simulink model "model_compatible"  (Simulink 7.5)
(part 10 of 10)

  T_173659686_220000_Enichem_Ottana/RConn1 -- L_173659686/LConn1
  T_173659686_220000_Enichem_Ottana/RConn2 -- L_173659686/LConn2
  L_173659686/LConn3 -- T_173659686_220000_Enichem_Ottana/RConn3 -- bus504/LConn1
  T_144006711_220000_Ottana/RConn1 -- L_144006711/LConn1
  T_144006711_220000_Ottana/RConn2 -- L_144006711/LConn2
  L_144006711/LConn3 -- T_144006711_220000_Ottana/RConn3 -- bus505/LConn1
  T_41360305_380000_Poggio_a_Caiano/RConn1 -- L_41360305/LConn1
  T_41360305_380000_Poggio_a_Caiano/RConn2 -- L_41360305/LConn2
  L_41360305/LConn3 -- T_41360305_380000_Poggio_a_Caiano/RConn3 -- bus506/LConn1
  T_139975773_380000_Casellina/RConn1 -- L_139975773/LConn1
  T_139975773_380000_Casellina/RConn2 -- L_139975773/LConn2
  L_139975773/LConn3 -- T_139975773_380000_Casellina/RConn3 -- bus507/LConn1
  T_132455976_220000_Sant'Antimo/RConn1 -- L_132455976/LConn1
  T_132455976_220000_Sant'Antimo/RConn2 -- L_132455976/LConn2
  L_132455976/LConn3 -- T_132455976_220000_Sant'Antimo/RConn3 -- bus508/LConn1
  T_132725149_220000_Astroni/RConn1 -- L_132725149/LConn1
  T_132725149_220000_Astroni/RConn2 -- L_132725149/LConn2
  L_132725149/LConn3 -- T_132725149_220000_Astroni/RConn3 -- bus509/LConn1
  T_132702940_60000;220000_Frattamaggiore/RConn1 -- L_132702940/LConn1
  T_132702940_60000;220000_Frattamaggiore/RConn2 -- L_132702940/LConn2
  L_132702940/LConn3 -- T_132702940_60000;220000_Frattamaggiore/RConn3 -- bus510/LConn1
  T_36873258_380000_Candia/RConn1 -- L_36873258/LConn1
  T_36873258_380000_Candia/RConn2 -- L_36873258/LConn2
  L_36873258/LConn3 -- T_36873258_380000_Candia/RConn3 -- bus511/LConn1
  T_136457747_220000_Abbadia/RConn1 -- L_136457747/LConn1
  T_136457747_220000_Abbadia/RConn2 -- L_136457747/LConn2
  L_136457747/LConn3 -- T_136457747_220000_Abbadia/RConn3 -- bus512/LConn1
  T_158652469_220000_Montorio/RConn1 -- L_158652469/LConn1
  T_158652469_220000_Montorio/RConn2 -- L_158652469/LConn2
  L_158652469/LConn3 -- T_158652469_220000_Montorio/RConn3 -- bus513/LConn1
  T_159821869_220000_Soverzene/RConn1 -- L_159821869/LConn1
  T_159821869_220000_Soverzene/RConn2 -- L_159821869/LConn2
  L_159821869/LConn3 -- T_159821869_220000_Soverzene/RConn3 -- bus514/LConn1
  T_128602121_220000_Scorzè/RConn1 -- L_128602121/LConn1
  T_128602121_220000_Scorzè/RConn2 -- L_128602121/LConn2
  L_128602121/LConn3 -- T_128602121_220000_Scorzè/RConn3 -- bus515/LConn1
  T_155976582_220000_Fadalto/RConn1 -- L_155976582/LConn1
  T_155976582_220000_Fadalto/RConn2 -- L_155976582/LConn2
  L_155976582/LConn3 -- T_155976582_220000_Fadalto/RConn3 -- bus516/LConn1
  T_84963374_220000_Flaminia/RConn1 -- L_84963374/LConn1
  T_84963374_220000_Flaminia/RConn2 -- L_84963374/LConn2
  L_84963374/LConn3 -- T_84963374_220000_Flaminia/RConn3 -- bus517/LConn1
  T_165371026__/RConn1 -- L_165371026/LConn1
  T_165371026__/RConn2 -- L_165371026/LConn2
  L_165371026/LConn3 -- T_165371026__/RConn3 -- bus518/LConn1
  T_105827045_220000_Sant'Antonio/RConn1 -- L_105827045/LConn1
  T_105827045_220000_Sant'Antonio/RConn2 -- L_105827045/LConn2
  L_105827045/LConn3 -- T_105827045_220000_Sant'Antonio/RConn3 -- bus519/LConn1
  T_105801489_220000_Kardaun___Cardano/RConn1 -- L_105801489/LConn1
  T_105801489_220000_Kardaun___Cardano/RConn2 -- L_105801489/LConn2
  L_105801489/LConn3 -- T_105801489_220000_Kardaun___Cardano/RConn3 -- bus520/LConn1
  T_147466201_220000_Santa_Massenza_Centrale/RConn1 -- L_147466201/LConn1
  T_147466201_220000_Santa_Massenza_Centrale/RConn2 -- L_147466201/LConn2
  L_147466201/LConn3 -- T_147466201_220000_Santa_Massenza_Centrale/RConn3 -- bus521/LConn1
  T_166196787_220000_Dalmine_BG/RConn1 -- L_166196787/LConn1
  T_166196787_220000_Dalmine_BG/RConn2 -- L_166196787/LConn2
  L_166196787/LConn3 -- T_166196787_220000_Dalmine_BG/RConn3 -- bus522/LConn1
  T_75378894_380000_Cislago/RConn1 -- L_75378894/LConn1
  T_75378894_380000_Cislago/RConn2 -- L_75378894/LConn2
  L_75378894/LConn3 -- T_75378894_380000_Cislago/RConn3 -- bus523/LConn1
  T_68299044_380000_Brugherio___Smistamento_elettrico_TERNA/RConn1 -- L_68299044/LConn1
  T_68299044_380000_Brugherio___Smistamento_elettrico_TERNA/RConn2 -- L_68299044/LConn2
  L_68299044/LConn3 -- T_68299044_380000_Brugherio___Smistamento_elettrico_TERNA/RConn3 -- bus524/LConn1
  T_103264820_220000_Magenta/RConn1 -- L_103264820/LConn1
  T_103264820_220000_Magenta/RConn2 -- L_103264820/LConn2
  L_103264820/LConn3 -- T_103264820_220000_Magenta/RConn3 -- bus525/LConn1
  T_67461115_220000_Novara_Sud/RConn1 -- L_67461115/LConn1
  T_67461115_220000_Novara_Sud/RConn2 -- L_67461115/LConn2
  L_67461115/LConn3 -- T_67461115_220000_Novara_Sud/RConn3 -- bus526/LConn1
  T_62326314_380000_Baggio/RConn1 -- L_62326314/LConn1
  T_62326314_380000_Baggio/RConn2 -- L_62326314/LConn2
  L_62326314/LConn3 -- T_62326314_380000_Baggio/RConn3 -- bus527/LConn1
  T_104114052_220000_Pallanzeno_1/RConn1 -- L_104114052/LConn1
  T_104114052_220000_Pallanzeno_1/RConn2 -- L_104114052/LConn2
  L_104114052/LConn3 -- T_104114052_220000_Pallanzeno_1/RConn3 -- bus528/LConn1
  T_133601333_220000_Cassano_220/RConn1 -- L_133601333/LConn1
  T_133601333_220000_Cassano_220/RConn2 -- L_133601333/LConn2
  L_133601333/LConn3 -- T_133601333_220000_Cassano_220/RConn3 -- bus529/LConn1
  T_116692433_220000_Brescia_Ricevitrice_Ovest/RConn1 -- L_116692433/LConn1
  T_116692433_220000_Brescia_Ricevitrice_Ovest/RConn2 -- L_116692433/LConn2
  L_116692433/LConn3 -- T_116692433_220000_Brescia_Ricevitrice_Ovest/RConn3 -- bus530/LConn1
  T_135270825_220000_Ricevitrice_Sud_Milano/RConn1 -- L_135270825/LConn1
  T_135270825_220000_Ricevitrice_Sud_Milano/RConn2 -- L_135270825/LConn2
  L_135270825/LConn3 -- T_135270825_220000_Ricevitrice_Sud_Milano/RConn3 -- bus531/LConn1
  T_281091768__Malcontenta/RConn1 -- L_281091768/LConn1
  T_281091768__Malcontenta/RConn2 -- L_281091768/LConn2
  L_281091768/LConn3 -- T_281091768__Malcontenta/RConn3 -- bus532/LConn1
  T_202272734_220000_Castegnero/RConn1 -- L_202272734/LConn1
  T_202272734_220000_Castegnero/RConn2 -- L_202272734/LConn2
  L_202272734/LConn3 -- T_202272734_220000_Castegnero/RConn3 -- bus533/LConn1
  T_59153311_380000_Dolo/RConn1 -- L_59153311/LConn1
  T_59153311_380000_Dolo/RConn2 -- L_59153311/LConn2
  L_59153311/LConn3 -- T_59153311_380000_Dolo/RConn3 -- bus534/LConn1
  T_59026315_380000_Salgareda/RConn1 -- L_59026315/LConn1
  T_59026315_380000_Salgareda/RConn2 -- L_59026315/LConn2
  L_59026315/LConn3 -- T_59026315_380000_Salgareda/RConn3 -- bus535/LConn1
  T_59366523_380000;220000;132000_Stazione_elettrica_di_Camin/RConn4 -- L_59366523/LConn1
  T_59366523_380000;220000;132000_Stazione_elettrica_di_Camin/RConn5 -- L_59366523/LConn2
  L_59366523/LConn3 -- T_59366523_380000;220000;132000_Stazione_elettrica_di_Camin/RConn6 -- bus536/LConn1
  T_144005861_220000_Villasor_Centrale/RConn1 -- L_144005861/LConn1
  T_144005861_220000_Villasor_Centrale/RConn2 -- L_144005861/LConn2
  L_144005861/LConn3 -- T_144005861_220000_Villasor_Centrale/RConn3 -- bus537/LConn1
  T_375892276_220000_Portoscuso/RConn1 -- L_375892276/LConn1
  T_375892276_220000_Portoscuso/RConn2 -- L_375892276/LConn2
  L_375892276/LConn3 -- T_375892276_220000_Portoscuso/RConn3 -- bus538/LConn1
  T_57384507_380000_Chiaramonte_Gulfi/RConn1 -- L_57384507/LConn1
  T_57384507_380000_Chiaramonte_Gulfi/RConn2 -- L_57384507/LConn2
  L_57384507/LConn3 -- T_57384507_380000_Chiaramonte_Gulfi/RConn3 -- bus539/LConn1
  T_57380344_220000_Ragusa/RConn1 -- L_57380344/LConn1
  T_57380344_220000_Ragusa/RConn2 -- L_57380344/LConn2
  L_57380344/LConn3 -- T_57380344_220000_Ragusa/RConn3 -- bus540/LConn1
  T_56984450_220000_Favara/RConn1 -- L_56984450/LConn1
  T_56984450_220000_Favara/RConn2 -- L_56984450/LConn2
  L_56984450/LConn3 -- T_56984450_220000_Favara/RConn3 -- bus541/LConn1
  T_210352188_220000_Ghrighine_Centrale/RConn1 -- L_210352188/LConn1
  T_210352188_220000_Ghrighine_Centrale/RConn2 -- L_210352188/LConn2
  L_210352188/LConn3 -- T_210352188_220000_Ghrighine_Centrale/RConn3 -- bus542/LConn1
  T_210352180_220000_CenTrale_Tirso/RConn1 -- L_210352180/LConn1
  T_210352180_220000_CenTrale_Tirso/RConn2 -- L_210352180/LConn2
  L_210352180/LConn3 -- T_210352180_220000_CenTrale_Tirso/RConn3 -- bus543/LConn1
  T_85196861_380000_Montecorvino/RConn1 -- L_85196861/LConn1
  T_85196861_380000_Montecorvino/RConn2 -- L_85196861/LConn2
  L_85196861/LConn3 -- T_85196861_380000_Montecorvino/RConn3 -- bus544/LConn1
  T_376952616_220000_Nocera/RConn1 -- L_376952616/LConn1
  T_376952616_220000_Nocera/RConn2 -- L_376952616/LConn2
  L_376952616/LConn3 -- T_376952616_220000_Nocera/RConn3 -- bus545/LConn1
  T_124220303_220000_Salerno_Nord/RConn1 -- L_124220303/LConn1
  T_124220303_220000_Salerno_Nord/RConn2 -- L_124220303/LConn2
  L_124220303/LConn3 -- T_124220303_220000_Salerno_Nord/RConn3 -- bus546/LConn1
  T_420698910_220000_Tusciano/RConn1 -- L_420698910/LConn1
  T_420698910_220000_Tusciano/RConn2 -- L_420698910/LConn2
  L_420698910/LConn3 -- T_420698910_220000_Tusciano/RConn3 -- bus547/LConn1
  T_85297730_220000_Gragnano/RConn1 -- L_85297730/LConn1
  T_85297730_220000_Gragnano/RConn2 -- L_85297730/LConn2
  L_85297730/LConn3 -- T_85297730_220000_Gragnano/RConn3 -- bus548/LConn1
  T_147455038_220000_Santa_Massenza_Smistamento/RConn1 -- L_147455038/LConn1
  T_147455038_220000_Santa_Massenza_Smistamento/RConn2 -- L_147455038/LConn2
  L_147455038/LConn3 -- T_147455038_220000_Santa_Massenza_Smistamento/RConn3 -- bus549/LConn1
  T_156001963_220000_Stazione_elettrica_di_Sandrà/RConn1 -- L_156001963/LConn1
  T_156001963_220000_Stazione_elettrica_di_Sandrà/RConn2 -- L_156001963/LConn2
  L_156001963/LConn3 -- T_156001963_220000_Stazione_elettrica_di_Sandrà/RConn3 -- bus550/LConn1
  T_132638645_220000_Brusciano/RConn1 -- L_132638645/LConn1
  T_132638645_220000_Brusciano/RConn2 -- L_132638645/LConn2
  L_132638645/LConn3 -- T_132638645_220000_Brusciano/RConn3 -- bus551/LConn1
  T_202711181_220000_Nola/RConn1 -- L_202711181/LConn1
  T_202711181_220000_Nola/RConn2 -- L_202711181/LConn2
  L_202711181/LConn3 -- T_202711181_220000_Nola/RConn3 -- bus552/LConn1
  T_132637884_220000_Fiat_Auto/RConn1 -- L_132637884/LConn1
  T_132637884_220000_Fiat_Auto/RConn2 -- L_132637884/LConn2
  L_132637884/LConn3 -- T_132637884_220000_Fiat_Auto/RConn3 -- bus553/LConn1
  T_132638412__/RConn1 -- L_132638412/LConn1
  T_132638412__/RConn2 -- L_132638412/LConn2
  L_132638412/LConn3 -- T_132638412__/RConn3 -- bus554/LConn1
  T_132701023_220000_Acerra_smistamento/RConn1 -- L_132701023/LConn1
  T_132701023_220000_Acerra_smistamento/RConn2 -- L_132701023/LConn2
  L_132701023/LConn3 -- T_132701023_220000_Acerra_smistamento/RConn3 -- bus555/LConn1
  T_132717802_220000_Maddaloni/RConn1 -- L_132717802/LConn1
  T_132717802_220000_Maddaloni/RConn2 -- L_132717802/LConn2
  L_132717802/LConn3 -- T_132717802_220000_Maddaloni/RConn3 -- bus556/LConn1
  T_163789376_220000_Venina/RConn1 -- L_163789376/LConn1
  T_163789376_220000_Venina/RConn2 -- L_163789376/LConn2
  L_163789376/LConn3 -- T_163789376_220000_Venina/RConn3 -- bus557/LConn1
  T_75947658_220000_Cassano_CS/RConn1 -- L_75947658/LConn1
  T_75947658_220000_Cassano_CS/RConn2 -- L_75947658/LConn2
  L_75947658/LConn3 -- T_75947658_220000_Cassano_CS/RConn3 -- bus558/LConn1
  T_114659171_220000_/RConn1 -- L_114659171/LConn1
  T_114659171_220000_/RConn2 -- L_114659171/LConn2
  L_114659171/LConn3 -- T_114659171_220000_/RConn3 -- bus559/LConn1
  T_318173253__/RConn1 -- L_318173253/LConn1
  T_318173253__/RConn2 -- L_318173253/LConn2
  L_318173253/LConn3 -- T_318173253__/RConn3 -- bus560/LConn1
  T_163056526_220000_Lanzada/RConn1 -- L_163056526/LConn1
  T_163056526_220000_Lanzada/RConn2 -- L_163056526/LConn2
  L_163056526/LConn3 -- T_163056526_220000_Lanzada/RConn3 -- bus561/LConn1
  T_163056522_220000_Sondrio/RConn1 -- L_163056522/LConn1
  T_163056522_220000_Sondrio/RConn2 -- L_163056522/LConn2
  L_163056522/LConn3 -- T_163056522_220000_Sondrio/RConn3 -- bus562/LConn1
  T_59629638_220000_Erzelli/RConn1 -- L_59629638/LConn1
  T_59629638_220000_Erzelli/RConn2 -- L_59629638/LConn2
  L_59629638/LConn3 -- T_59629638_220000_Erzelli/RConn3 -- bus563/LConn1
  T_61484190_220000_Morigallo/RConn1 -- L_61484190/LConn1
  T_61484190_220000_Morigallo/RConn2 -- L_61484190/LConn2
  L_61484190/LConn3 -- T_61484190_220000_Morigallo/RConn3 -- bus564/LConn1
  T_376952589_220000_/RConn1 -- L_376952589/LConn1
  T_376952589_220000_/RConn2 -- L_376952589/LConn2
  L_376952589/LConn3 -- T_376952589_220000_/RConn3 -- bus565/LConn1
  T_370679021_220000_Casalnuovo/RConn1 -- L_370679021/LConn1
  T_370679021_220000_Casalnuovo/RConn2 -- L_370679021/LConn2
  L_370679021/LConn3 -- T_370679021_220000_Casalnuovo/RConn3 -- bus566/LConn1
  T_376952600_220000_Alfa_Avio/RConn1 -- L_376952600/LConn1
  T_376952600_220000_Alfa_Avio/RConn2 -- L_376952600/LConn2
  L_376952600/LConn3 -- T_376952600_220000_Alfa_Avio/RConn3 -- bus567/LConn1
  T_199886416_220000_Mercure/RConn1 -- L_199886416/LConn1
  T_199886416_220000_Mercure/RConn2 -- L_199886416/LConn2
  L_199886416/LConn3 -- T_199886416_220000_Mercure/RConn3 -- bus568/LConn1
  T_108020695_220000_Rotonda/RConn1 -- L_108020695/LConn1
  T_108020695_220000_Rotonda/RConn2 -- L_108020695/LConn2
  L_108020695/LConn3 -- T_108020695_220000_Rotonda/RConn3 -- bus569/LConn1
  T_129407370_220000_Stazione_IV/RConn1 -- L_129407370/LConn1
  T_129407370_220000_Stazione_IV/RConn2 -- L_129407370/LConn2
  L_129407370/LConn3 -- T_129407370_220000_Stazione_IV/RConn3 -- bus570/LConn1
  T_416679117_220000_Villabona/RConn1 -- L_416679117/LConn1
  T_416679117_220000_Villabona/RConn2 -- L_416679117/LConn2
  L_416679117/LConn3 -- T_416679117_220000_Villabona/RConn3 -- bus571/LConn1
  T_129406824_220000;132000_Azotati/RConn1 -- L_129406824/LConn1
  T_129406824_220000;132000_Azotati/RConn2 -- L_129406824/LConn2
  L_129406824/LConn3 -- T_129406824_220000;132000_Azotati/RConn3 -- bus572/LConn1
  T_61650514_220000_Somplago_centrale/RConn1 -- L_61650514/LConn1
  T_61650514_220000_Somplago_centrale/RConn2 -- L_61650514/LConn2
  L_61650514/LConn3 -- T_61650514_220000_Somplago_centrale/RConn3 -- bus573/LConn1
  T_149188707_220000_Cittadella/RConn1 -- L_149188707/LConn1
  T_149188707_220000_Cittadella/RConn2 -- L_149188707/LConn2
  L_149188707/LConn3 -- T_149188707_220000_Cittadella/RConn3 -- bus574/LConn1
  T_128523865_220000_Acciaierie_Venete_220/RConn1 -- L_128523865/LConn1
  T_128523865_220000_Acciaierie_Venete_220/RConn2 -- L_128523865/LConn2
  L_128523865/LConn3 -- T_128523865_220000_Acciaierie_Venete_220/RConn3 -- bus575/LConn1
  T_105062415_220000_Pianezza/RConn1 -- L_105062415/LConn1
  T_105062415_220000_Pianezza/RConn2 -- L_105062415/LConn2
  L_105062415/LConn3 -- T_105062415_220000_Pianezza/RConn3 -- bus576/LConn1
  T_58516664_220000_Martinetto/RConn1 -- L_58516664/LConn1
  T_58516664_220000_Martinetto/RConn2 -- L_58516664/LConn2
  L_58516664/LConn3 -- T_58516664_220000_Martinetto/RConn3 -- bus577/LConn1
  T_105141350_220000_Grugliasco/RConn1 -- L_105141350/LConn1
  T_105141350_220000_Grugliasco/RConn2 -- L_105141350/LConn2
  L_105141350/LConn3 -- T_105141350_220000_Grugliasco/RConn3 -- bus578/LConn1
  T_66872608_220000_Rosone/RConn1 -- L_66872608/LConn1
  T_66872608_220000_Rosone/RConn2 -- L_66872608/LConn2
  L_66872608/LConn3 -- T_66872608_220000_Rosone/RConn3 -- bus579/LConn1
  T_98902899_380000_Piossasco/RConn1 -- L_98902899/LConn1
  T_98902899_380000_Piossasco/RConn2 -- L_98902899/LConn2
  L_98902899/LConn3 -- T_98902899_380000_Piossasco/RConn3 -- bus580/LConn1
  T_163958919_220000_Lambrate/RConn1 -- L_163958919/LConn1
  T_163958919_220000_Lambrate/RConn2 -- L_163958919/LConn2
  L_163958919/LConn3 -- T_163958919_220000_Lambrate/RConn3 -- bus581/LConn1
  T_203771704_220000_UT_CESI/RConn1 -- L_203771704/LConn1
  T_203771704_220000_UT_CESI/RConn2 -- L_203771704/LConn2
  L_203771704/LConn3 -- T_203771704_220000_UT_CESI/RConn3 -- bus582/LConn1
  T_173999201_220000_Napoli_Levante/RConn1 -- L_173999201/LConn1
  T_173999201_220000_Napoli_Levante/RConn2 -- L_173999201/LConn2
  L_173999201/LConn3 -- T_173999201_220000_Napoli_Levante/RConn3 -- bus583/LConn1
  T_376502734_220000_Casoria/RConn1 -- L_376502734/LConn1
  T_376502734_220000_Casoria/RConn2 -- L_376502734/LConn2
  L_376502734/LConn3 -- T_376502734_220000_Casoria/RConn3 -- bus584/LConn1
  T_377444648_220000_/RConn1 -- L_377444648/LConn1
  T_377444648_220000_/RConn2 -- L_377444648/LConn2
  L_377444648/LConn3 -- T_377444648_220000_/RConn3 -- bus585/LConn1
  T_80442466_220000_Grosio/RConn1 -- L_80442466/LConn1
  T_80442466_220000_Grosio/RConn2 -- L_80442466/LConn2
  L_80442466/LConn3 -- T_80442466_220000_Grosio/RConn3 -- bus586/LConn1
  T_165503884_220000_Grosotto/RConn1 -- L_165503884/LConn1
  T_165503884_220000_Grosotto/RConn2 -- L_165503884/LConn2
  L_165503884/LConn3 -- T_165503884_220000_Grosotto/RConn3 -- bus587/LConn1
  T_105757795_220000_Campochiesa/RConn1 -- L_105757795/LConn1
  T_105757795_220000_Campochiesa/RConn2 -- L_105757795/LConn2
  L_105757795/LConn3 -- T_105757795_220000_Campochiesa/RConn3 -- bus588/LConn1
  T_103653567_220000_centrale_elettrica_di_Camporosso/RConn1 -- L_103653567/LConn1
  T_103653567_220000_centrale_elettrica_di_Camporosso/RConn2 -- L_103653567/LConn2
  L_103653567/LConn3 -- T_103653567_220000_centrale_elettrica_di_Camporosso/RConn3 -- bus589/LConn1
  T_309371153_220000_TO_Sud/RConn1 -- L_309371153/LConn1
  T_309371153_220000_TO_Sud/RConn2 -- L_309371153/LConn2
  L_309371153/LConn3 -- T_309371153_220000_TO_Sud/RConn3 -- bus590/LConn1
  T_309371152_220000_TO_Centro/RConn1 -- L_309371152/LConn1
  T_309371152_220000_TO_Centro/RConn2 -- L_309371152/LConn2
  L_309371152/LConn3 -- T_309371152_220000_TO_Centro/RConn3 -- bus591/LConn1
  T_350356755_220000_Colorno/RConn1 -- L_350356755/LConn1
  T_350356755_220000_Colorno/RConn2 -- L_350356755/LConn2
  L_350356755/LConn3 -- T_350356755_220000_Colorno/RConn3 -- bus592/LConn1
  T_163058980_220000_Marcaria/RConn1 -- L_163058980/LConn1
  T_163058980_220000_Marcaria/RConn2 -- L_163058980/LConn2
  L_163058980/LConn3 -- T_163058980_220000_Marcaria/RConn3 -- bus593/LConn1
  T_191960170_220000_Corriolo/RConn1 -- L_191960170/LConn1
  T_191960170_220000_Corriolo/RConn2 -- L_191960170/LConn2
  L_191960170/LConn3 -- T_191960170_220000_Corriolo/RConn3 -- bus594/LConn1
  T_57736553_220000_Caracoli/RConn1 -- L_57736553/LConn1
  T_57736553_220000_Caracoli/RConn2 -- L_57736553/LConn2
  L_57736553/LConn3 -- T_57736553_220000_Caracoli/RConn3 -- bus595/LConn1
  T_136626367__/RConn1 -- L_136626367/LConn1
  T_136626367__/RConn2 -- L_136626367/LConn2
  L_136626367/LConn3 -- T_136626367__/RConn3 -- bus596/LConn1
  T_375892275_220000_Eurallumina/RConn1 -- L_375892275/LConn1
  T_375892275_220000_Eurallumina/RConn2 -- L_375892275/LConn2
  L_375892275/LConn3 -- T_375892275_220000_Eurallumina/RConn3 -- bus597/LConn1
  T_375892277_220000_Samim/RConn1 -- L_375892277/LConn1
  T_375892277_220000_Samim/RConn2 -- L_375892277/LConn2
  L_375892277/LConn3 -- T_375892277_220000_Samim/RConn3 -- bus598/LConn1
  T_375892272_220000_Samim/RConn1 -- L_375892272/LConn1
  T_375892272_220000_Samim/RConn2 -- L_375892272/LConn2
  L_375892272/LConn3 -- T_375892272_220000_Samim/RConn3 -- bus599/LConn1
  T_107204719_220000_Tavazzano_Est/RConn1 -- L_107204719/LConn1
  T_107204719_220000_Tavazzano_Est/RConn2 -- L_107204719/LConn2
  L_107204719/LConn3 -- T_107204719_220000_Tavazzano_Est/RConn3 -- bus600/LConn1
  T_74359510_220000_Cesano_Maderno/RConn1 -- L_74359510/LConn1
  T_74359510_220000_Cesano_Maderno/RConn2 -- L_74359510/LConn2
  L_74359510/LConn3 -- T_74359510_220000_Cesano_Maderno/RConn3 -- bus601/LConn1
  T_156001981_220000_Colà/RConn1 -- L_156001981/LConn1
  T_156001981_220000_Colà/RConn2 -- L_156001981/LConn2
  L_156001981/LConn3 -- T_156001981_220000_Colà/RConn3 -- bus602/LConn1
  T_116916459_220000_Tavazzano_ST/RConn1 -- L_116916459/LConn1
  T_116916459_220000_Tavazzano_ST/RConn2 -- L_116916459/LConn2
  L_116916459/LConn3 -- T_116916459_220000_Tavazzano_ST/RConn3 -- bus603/LConn1
  T_60725872_380000_Monfalcone_sezione_1_220/LConn1 -- L_60725872/LConn1
  T_60725872_380000_Monfalcone_sezione_1_220/LConn2 -- L_60725872/LConn2
  L_60725872/LConn3 -- T_60725872_380000_Monfalcone_sezione_1_220/LConn3 -- bus604/LConn1
  T_41892273_380000_Redipuglia/RConn1 -- L_41892273/LConn1
  T_41892273_380000_Redipuglia/RConn2 -- L_41892273/LConn2
  L_41892273/LConn3 -- T_41892273_380000_Redipuglia/RConn3 -- bus605/LConn1
  T_61038773_220000_Padriciano/RConn1 -- L_61038773/LConn1
  T_61038773_220000_Padriciano/RConn2 -- L_61038773/LConn2
  L_61038773/LConn3 -- T_61038773_220000_Padriciano/RConn3 -- bus606/LConn1
  T_105141365_380000_Laboratori_Cesi_Chivasso/RConn1 -- L_105141365/LConn1
  T_105141365_380000_Laboratori_Cesi_Chivasso/RConn2 -- L_105141365/LConn2
  L_105141365/LConn3 -- T_105141365_380000_Laboratori_Cesi_Chivasso/RConn3 -- bus607/LConn1
  T_82651599_220000_Biella_Est/RConn1 -- L_82651599/LConn1
  T_82651599_220000_Biella_Est/RConn2 -- L_82651599/LConn2
  L_82651599/LConn3 -- T_82651599_220000_Biella_Est/RConn3 -- bus608/LConn1
  T_74869121_380000_Rondissone/RConn1 -- L_74869121/LConn1
  T_74869121_380000_Rondissone/RConn2 -- L_74869121/LConn2
  L_74869121/LConn3 -- T_74869121_380000_Rondissone/RConn3 -- bus609/LConn1
  T_103725268_220000_Stura/RConn1 -- L_103725268/LConn1
  T_103725268_220000_Stura/RConn2 -- L_103725268/LConn2
  L_103725268/LConn3 -- T_103725268_220000_Stura/RConn3 -- bus610/LConn1
  T_100952845_380000_Vignole/RConn1 -- L_100952845/LConn1
  T_100952845_380000_Vignole/RConn2 -- L_100952845/LConn2
  L_100952845/LConn3 -- T_100952845_380000_Vignole/RConn3 -- bus611/LConn1
  T_79879290_220000_Ricevitrice_Nord_Milano/RConn1 -- L_79879290/LConn1
  T_79879290_220000_Ricevitrice_Nord_Milano/RConn2 -- L_79879290/LConn2
  L_79879290/LConn3 -- T_79879290_220000_Ricevitrice_Nord_Milano/RConn3 -- bus612/LConn1
  T_146652798_220000_Centro_Energia_Teverola/RConn1 -- L_146652798/LConn1
  T_146652798_220000_Centro_Energia_Teverola/RConn2 -- L_146652798/LConn2
  L_146652798/LConn3 -- T_146652798_220000_Centro_Energia_Teverola/RConn3 -- bus613/LConn1
  T_132701980_220000_Aversa/RConn1 -- L_132701980/LConn1
  T_132701980_220000_Aversa/RConn2 -- L_132701980/LConn2
  L_132701980/LConn3 -- T_132701980_220000_Aversa/RConn3 -- bus614/LConn1
  T_96658563_220000_Lavis/RConn1 -- L_96658563/LConn1
  T_96658563_220000_Lavis/RConn2 -- L_96658563/LConn2
  L_96658563/LConn3 -- T_96658563_220000_Lavis/RConn3 -- bus615/LConn1
  T_103549584_220000_Borgo_Valsugana/RConn1 -- L_103549584/LConn1
  T_103549584_220000_Borgo_Valsugana/RConn2 -- L_103549584/LConn2
  L_103549584/LConn3 -- T_103549584_220000_Borgo_Valsugana/RConn3 -- bus616/LConn1
  T_151070909_220000_San_Floriano_d'Egna/RConn1 -- L_151070909/LConn1
  T_151070909_220000_San_Floriano_d'Egna/RConn2 -- L_151070909/LConn2
  L_151070909/LConn3 -- T_151070909_220000_San_Floriano_d'Egna/RConn3 -- bus617/LConn1
  T_419423704_220000_Presenzano_TR/RConn1 -- L_419423704/LConn1
  T_419423704_220000_Presenzano_TR/RConn2 -- L_419423704/LConn2
  L_419423704/LConn3 -- T_419423704_220000_Presenzano_TR/RConn3 -- bus618/LConn1
  T_93860115_380000_Santa_Maria_Capua_Vetere/RConn1 -- L_93860115/LConn1
  T_93860115_380000_Santa_Maria_Capua_Vetere/RConn2 -- L_93860115/LConn2
  L_93860115/LConn3 -- T_93860115_380000_Santa_Maria_Capua_Vetere/RConn3 -- bus619/LConn1
  T_202772821_220000_Ganda/RConn1 -- L_202772821/LConn1
  T_202772821_220000_Ganda/RConn2 -- L_202772821/LConn2
  L_202772821/LConn3 -- T_202772821_220000_Ganda/RConn3 -- bus620/LConn1
  T_61375111_380000_Villanova/RConn1 -- L_61375111/LConn1
  T_61375111_380000_Villanova/RConn2 -- L_61375111/LConn2
  L_61375111/LConn3 -- T_61375111_380000_Villanova/RConn3 -- bus621/LConn1
  T_139758444_220000_Querceto/RConn1 -- L_139758444/LConn1
  T_139758444_220000_Querceto/RConn2 -- L_139758444/LConn2
  L_139758444/LConn3 -- T_139758444_220000_Querceto/RConn3 -- bus622/LConn1
  T_139442467_380000_Colunga/RConn1 -- L_139442467/LConn1
  T_139442467_380000_Colunga/RConn2 -- L_139442467/LConn2
  L_139442467/LConn3 -- T_139442467_380000_Colunga/RConn3 -- bus623/LConn1
  T_40634284_380000_Calenzano/RConn1 -- L_40634284/LConn1
  T_40634284_380000_Calenzano/RConn2 -- L_40634284/LConn2
  L_40634284/LConn3 -- T_40634284_380000_Calenzano/RConn3 -- bus624/LConn1
  T_107241327_220000_Tavazzano_Ovest/RConn1 -- L_107241327/LConn1
  T_107241327_220000_Tavazzano_Ovest/RConn2 -- L_107241327/LConn2
  L_107241327/LConn3 -- T_107241327_220000_Tavazzano_Ovest/RConn3 -- bus625/LConn1
  T_203468251_220000;132000_RISE_Sesto/RConn1 -- L_203468251/LConn1
  T_203468251_220000;132000_RISE_Sesto/RConn2 -- L_203468251/LConn2
  L_203468251/LConn3 -- T_203468251_220000;132000_RISE_Sesto/RConn3 -- bus626/LConn1
  T_93850768_220000_Castelluccia/RConn1 -- L_93850768/LConn1
  T_93850768_220000_Castelluccia/RConn2 -- L_93850768/LConn2
  L_93850768/LConn3 -- T_93850768_220000_Castelluccia/RConn3 -- bus627/LConn1
  T_202179289_220000_/RConn1 -- L_202179289/LConn1
  T_202179289_220000_/RConn2 -- L_202179289/LConn2
  L_202179289/LConn3 -- T_202179289_220000_/RConn3 -- bus628/LConn1
  T_59604857_220000_Acciaieria_Bertoli/RConn1 -- L_59604857/LConn1
  T_59604857_220000_Acciaieria_Bertoli/RConn2 -- L_59604857/LConn2
  L_59604857/LConn3 -- T_59604857_220000_Acciaieria_Bertoli/RConn3 -- bus629/LConn1
  T_165371027__/RConn1 -- L_165371027/LConn1
  T_165371027__/RConn2 -- L_165371027/LConn2
  L_165371027/LConn3 -- T_165371027__/RConn3 -- bus630/LConn1
  T_82762493_380000_Santa_Lucia/RConn1 -- L_82762493/LConn1
  T_82762493_380000_Santa_Lucia/RConn2 -- L_82762493/LConn2
  L_82762493/LConn3 -- T_82762493_380000_Santa_Lucia/RConn3 -- bus631/LConn1
  T_151205012_220000_Boazzo/RConn1 -- L_151205012/LConn1
  T_151205012_220000_Boazzo/RConn2 -- L_151205012/LConn2
  L_151205012/LConn3 -- T_151205012_220000_Boazzo/RConn3 -- bus632/LConn1
  T_151199514_220000_Cimego_TR/RConn1 -- L_151199514/LConn1
  T_151199514_220000_Cimego_TR/RConn2 -- L_151199514/LConn2
  L_151199514/LConn3 -- T_151199514_220000_Cimego_TR/RConn3 -- bus633/LConn1
  T_103653565_220000_San_Colombano/RConn1 -- L_103653565/LConn1
  T_103653565_220000_San_Colombano/RConn2 -- L_103653565/LConn2
  L_103653565/LConn3 -- T_103653565_220000_San_Colombano/RConn3 -- bus634/LConn1
  T_158599954_220000_Stazione_elettrica_di_Avenza/RConn1 -- L_158599954/LConn1
  T_158599954_220000_Stazione_elettrica_di_Avenza/RConn2 -- L_158599954/LConn2
  L_158599954/LConn3 -- T_158599954_220000_Stazione_elettrica_di_Avenza/RConn3 -- bus635/LConn1
  T_296141722_220000_Savona_T5/RConn1 -- L_296141722/LConn1
  T_296141722_220000_Savona_T5/RConn2 -- L_296141722/LConn2
  L_296141722/LConn3 -- T_296141722_220000_Savona_T5/RConn3 -- bus636/LConn1
  T_375908008_220000_Fulgatore/RConn1 -- L_375908008/LConn1
  T_375908008_220000_Fulgatore/RConn2 -- L_375908008/LConn2
  L_375908008/LConn3 -- T_375908008_220000_Fulgatore/RConn3 -- bus637/LConn1
  T_53635045__Partanna/RConn1 -- L_53635045/LConn1
  T_53635045__Partanna/RConn2 -- L_53635045/LConn2
  L_53635045/LConn3 -- T_53635045__Partanna/RConn3 -- bus638/LConn1
  T_110140586_220000_San_Filippo_del_Mela_gruppi_5_e_6/RConn1 -- L_110140586/LConn1
  T_110140586_220000_San_Filippo_del_Mela_gruppi_5_e_6/RConn2 -- L_110140586/LConn2
  L_110140586/LConn3 -- T_110140586_220000_San_Filippo_del_Mela_gruppi_5_e_6/RConn3 -- bus639/LConn1
  T_111020792_220000_Stazione_elettrica_di_Bussolengo/RConn1 -- L_111020792/LConn1
  T_111020792_220000_Stazione_elettrica_di_Bussolengo/RConn2 -- L_111020792/LConn2
  L_111020792/LConn3 -- T_111020792_220000_Stazione_elettrica_di_Bussolengo/RConn3 -- bus640/LConn1
  T_59556712_380000_Dugale/RConn1 -- L_59556712/LConn1
  T_59556712_380000_Dugale/RConn2 -- L_59556712/LConn2
  L_59556712/LConn3 -- T_59556712_380000_Dugale/RConn3 -- bus641/LConn1
  T_412909650_220000_Mantova_220/RConn1 -- L_412909650/LConn1
  T_412909650_220000_Mantova_220/RConn2 -- L_412909650/LConn2
  L_412909650/LConn3 -- T_412909650_220000_Mantova_220/RConn3 -- bus642/LConn1
  T_155976563_220000_Conegliano/RConn1 -- L_155976563/LConn1
  T_155976563_220000_Conegliano/RConn2 -- L_155976563/LConn2
  L_155976563/LConn3 -- T_155976563_220000_Conegliano/RConn3 -- bus643/LConn1
  T_96188601_220000_San_Giacomo_220/RConn1 -- L_96188601/LConn1
  T_96188601_220000_San_Giacomo_220/RConn2 -- L_96188601/LConn2
  L_96188601/LConn3 -- T_96188601_220000_San_Giacomo_220/RConn3 -- bus644/LConn1
  T_84277460_220000_Popoli/RConn1 -- L_84277460/LConn1
  T_84277460_220000_Popoli/RConn2 -- L_84277460/LConn2
  L_84277460/LConn3 -- T_84277460_220000_Popoli/RConn3 -- bus645/LConn1
  T_96190189_380000_San_Giacomo_380/RConn1 -- L_96190189/LConn1
  T_96190189_380000_San_Giacomo_380/RConn2 -- L_96190189/LConn2
  L_96190189/LConn3 -- T_96190189_380000_San_Giacomo_380/RConn3 -- bus646/LConn1
  T_108020416_380000_Laino/RConn1 -- L_108020416/LConn1
  T_108020416_380000_Laino/RConn2 -- L_108020416/LConn2
  L_108020416/LConn3 -- T_108020416_380000_Laino/RConn3 -- bus647/LConn1
  T_144378054_220000_Arezzo_C/RConn1 -- L_144378054/LConn1
  T_144378054_220000_Arezzo_C/RConn2 -- L_144378054/LConn2
  L_144378054/LConn3 -- T_144378054_220000_Arezzo_C/RConn3 -- bus648/LConn1
  T_120916823_220000_Pietrafitta_220/RConn1 -- L_120916823/LConn1
  T_120916823_220000_Pietrafitta_220/RConn2 -- L_120916823/LConn2
  L_120916823/LConn3 -- T_120916823_220000_Pietrafitta_220/RConn3 -- bus649/LConn1
  T_59620552_220000_Naturno/RConn1 -- L_59620552/LConn1
  T_59620552_220000_Naturno/RConn2 -- L_59620552/LConn2
  L_59620552/LConn3 -- T_59620552_220000_Naturno/RConn3 -- bus650/LConn1
  T_35680992_220000_Ponte_Resia/RConn1 -- L_35680992/LConn1
  T_35680992_220000_Ponte_Resia/RConn2 -- L_35680992/LConn2
  L_35680992/LConn3 -- T_35680992_220000_Ponte_Resia/RConn3 -- bus651/LConn1
  T_101346507_220000_Novi_Ligure/RConn1 -- L_101346507/LConn1
  T_101346507_220000_Novi_Ligure/RConn2 -- L_101346507/LConn2
  L_101346507/LConn3 -- T_101346507_220000_Novi_Ligure/RConn3 -- bus652/LConn1
  T_101346508_220000_Ital_Novi/RConn1 -- L_101346508/LConn1
  T_101346508_220000_Ital_Novi/RConn2 -- L_101346508/LConn2
  L_101346508/LConn3 -- T_101346508_220000_Ital_Novi/RConn3 -- bus653/LConn1
  T_95466193_220000_/RConn1 -- L_95466193/LConn1
  T_95466193_220000_/RConn2 -- L_95466193/LConn2
  L_95466193/LConn3 -- T_95466193_220000_/RConn3 -- bus654/LConn1
  T_76705565_380000;220000;150000_Roma_Sud/RConn4 -- L_76705565/LConn1
  T_76705565_380000;220000;150000_Roma_Sud/RConn5 -- L_76705565/LConn2
  L_76705565/LConn3 -- T_76705565_380000;220000;150000_Roma_Sud/RConn6 -- bus655/LConn1
  T_375916035_220000_Cattolica_Eraclea_centrale/RConn1 -- L_375916035/LConn1
  T_375916035_220000_Cattolica_Eraclea_centrale/RConn2 -- L_375916035/LConn2
  L_375916035/LConn3 -- T_375916035_220000_Cattolica_Eraclea_centrale/RConn3 -- bus656/LConn1
  T_375907988_220000_Sambuca/RConn1 -- L_375907988/LConn1
  T_375907988_220000_Sambuca/RConn2 -- L_375907988/LConn2
  L_375907988/LConn3 -- T_375907988_220000_Sambuca/RConn3 -- bus657/LConn1
  T_132726160_220000_Pozzuoli/RConn1 -- L_132726160/LConn1
  T_132726160_220000_Pozzuoli/RConn2 -- L_132726160/LConn2
  L_132726160/LConn3 -- T_132726160_220000_Pozzuoli/RConn3 -- bus658/LConn1
  T_377832777_220000_Tirano/RConn1 -- L_377832777/LConn1
  T_377832777_220000_Tirano/RConn2 -- L_377832777/LConn2
  L_377832777/LConn3 -- T_377832777_220000_Tirano/RConn3 -- bus659/LConn1
  T_98787157_220000_Glorenza/RConn1 -- L_98787157/LConn1
  T_98787157_220000_Glorenza/RConn2 -- L_98787157/LConn2
  L_98787157/LConn3 -- T_98787157_220000_Glorenza/RConn3 -- bus660/LConn1
  T_377588184_220000_Caivano/RConn1 -- L_377588184/LConn1
  T_377588184_220000_Caivano/RConn2 -- L_377588184/LConn2
  L_377588184/LConn3 -- T_377588184_220000_Caivano/RConn3 -- bus661/LConn1
  T_132719324_220000_Air_Liquide/RConn1 -- L_132719324/LConn1
  T_132719324_220000_Air_Liquide/RConn2 -- L_132719324/LConn2
  L_132719324/LConn3 -- T_132719324_220000_Air_Liquide/RConn3 -- bus662/LConn1
  T_84696559_380000_Santa_Sofia/RConn1 -- L_84696559/LConn1
  T_84696559_380000_Santa_Sofia/RConn2 -- L_84696559/LConn2
  L_84696559/LConn3 -- T_84696559_380000_Santa_Sofia/RConn3 -- bus663/LConn1
  T_162960205_380000_Tavazzano_Centrale/RConn1 -- L_162960205/LConn1
  T_162960205_380000_Tavazzano_Centrale/RConn2 -- L_162960205/LConn2
  L_162960205/LConn3 -- T_162960205_380000_Tavazzano_Centrale/RConn3 -- bus664/LConn1
  T_214294769_220000_Moline/RConn1 -- L_214294769/LConn1
  T_214294769_220000_Moline/RConn2 -- L_214294769/LConn2
  L_214294769/LConn3 -- T_214294769_220000_Moline/RConn3 -- bus665/LConn1
  T_281837810_220000_Cedegolo_Sud/RConn1 -- L_281837810/LConn1
  T_281837810_220000_Cedegolo_Sud/RConn2 -- L_281837810/LConn2
  L_281837810/LConn3 -- T_281837810_220000_Cedegolo_Sud/RConn3 -- bus666/LConn1
  T_181125039_220000_Enipower_Ferrara/RConn1 -- L_181125039/LConn1
  T_181125039_220000_Enipower_Ferrara/RConn2 -- L_181125039/LConn2
  L_181125039/LConn3 -- T_181125039_220000_Enipower_Ferrara/RConn3 -- bus667/LConn1
  T_82078641_380000_Ostiglia/RConn1 -- L_82078641/LConn1
  T_82078641_380000_Ostiglia/RConn2 -- L_82078641/LConn2
  L_82078641/LConn3 -- T_82078641_380000_Ostiglia/RConn3 -- bus668/LConn1
  T_162066058_220000_Verona_Borgomilano/RConn1 -- L_162066058/LConn1
  T_162066058_220000_Verona_Borgomilano/RConn2 -- L_162066058/LConn2
  L_162066058/LConn3 -- T_162066058_220000_Verona_Borgomilano/RConn3 -- bus669/LConn1
  T_289178949_220000_Riva_Acciaio/RConn1 -- L_289178949/LConn1
  T_289178949_220000_Riva_Acciaio/RConn2 -- L_289178949/LConn2
  L_289178949/LConn3 -- T_289178949_220000_Riva_Acciaio/RConn3 -- bus670/LConn1
  T_103725446_220000_Sondel_Settimo_Torinese/RConn1 -- L_103725446/LConn1
  T_103725446_220000_Sondel_Settimo_Torinese/RConn2 -- L_103725446/LConn2
  L_103725446/LConn3 -- T_103725446_220000_Sondel_Settimo_Torinese/RConn3 -- bus671/LConn1
  T_82767145_380000_Tirreno_Power_Torrevaldaliga/RConn1 -- L_82767145/LConn1
  T_82767145_380000_Tirreno_Power_Torrevaldaliga/RConn2 -- L_82767145/LConn2
  L_82767145/LConn3 -- T_82767145_380000_Tirreno_Power_Torrevaldaliga/RConn3 -- bus672/LConn1
  T_194186027_220000_Duferdofin/RConn1 -- L_194186027/LConn1
  T_194186027_220000_Duferdofin/RConn2 -- L_194186027/LConn2
  L_194186027/LConn3 -- T_194186027_220000_Duferdofin/RConn3 -- bus673/LConn1
  T_338948868_220000_Termini_Centrale_gruppi_6/RConn1 -- L_338948868/LConn1
  T_338948868_220000_Termini_Centrale_gruppi_6/RConn2 -- L_338948868/LConn2
  L_338948868/LConn3 -- T_338948868_220000_Termini_Centrale_gruppi_6/RConn3 -- bus674/LConn1
  T_145665797_220000_Brindisi_Nord_220/RConn1 -- L_145665797/LConn1
  T_145665797_220000_Brindisi_Nord_220/RConn2 -- L_145665797/LConn2
  L_145665797/LConn3 -- T_145665797_220000_Brindisi_Nord_220/RConn3 -- bus675/LConn1
  T_103653591_220000_Vado_Stazione/RConn1 -- L_103653591/LConn1
  T_103653591_220000_Vado_Stazione/RConn2 -- L_103653591/LConn2
  L_103653591/LConn3 -- T_103653591_220000_Vado_Stazione/RConn3 -- bus676/LConn1
  T_100407576_380000_Fusina_Termica_sezione_1_220/LConn1 -- L_100407576/LConn1
  T_100407576_380000_Fusina_Termica_sezione_1_220/LConn2 -- L_100407576/LConn2
  L_100407576/LConn3 -- T_100407576_380000_Fusina_Termica_sezione_1_220/LConn3 -- bus677/LConn1
  T_95466377_220000_/RConn1 -- L_95466377/LConn1
  T_95466377_220000_/RConn2 -- L_95466377/LConn2
  L_95466377/LConn3 -- T_95466377_220000_/RConn3 -- bus678/LConn1
  T_102185356_220000_Villa/RConn1 -- L_102185356/LConn1
  T_102185356_220000_Villa/RConn2 -- L_102185356/LConn2
  L_102185356/LConn3 -- T_102185356_220000_Villa/RConn3 -- bus679/LConn1
  T_162828577_380000_Turbigo/RConn1 -- L_162828577/LConn1
  T_162828577_380000_Turbigo/RConn2 -- L_162828577/LConn2
  L_162828577/LConn3 -- T_162828577_380000_Turbigo/RConn3 -- bus680/LConn1
  T_136708548_220000_Certosa/RConn1 -- L_136708548/LConn1
  T_136708548_220000_Certosa/RConn2 -- L_136708548/LConn2
  L_136708548/LConn3 -- T_136708548_220000_Certosa/RConn3 -- bus681/LConn1
  T_118987056_380000_Selargius/RConn1 -- L_118987056/LConn1
  T_118987056_380000_Selargius/RConn2 -- L_118987056/LConn2
  L_118987056/LConn3 -- T_118987056_380000_Selargius/RConn3 -- bus682/LConn1
  T_377444657_220000_Secondigliano/RConn1 -- L_377444657/LConn1
  T_377444657_220000_Secondigliano/RConn2 -- L_377444657/LConn2
  L_377444657/LConn3 -- T_377444657_220000_Secondigliano/RConn3 -- bus683/LConn1
  T_172705586__Bellolampo/RConn1 -- L_172705586/LConn1
  T_172705586__Bellolampo/RConn2 -- L_172705586/LConn2
  L_172705586/LConn3 -- T_172705586__Bellolampo/RConn3 -- bus684/LConn1
  T_57736541__Partinico/RConn1 -- L_57736541/LConn1
  T_57736541__Partinico/RConn2 -- L_57736541/LConn2
  L_57736541/LConn3 -- T_57736541__Partinico/RConn3 -- bus685/LConn1
  T_103007030_220000_Chatillon_Centrale/RConn1 -- L_103007030/LConn1
  T_103007030_220000_Chatillon_Centrale/RConn2 -- L_103007030/LConn2
  L_103007030/LConn3 -- T_103007030_220000_Chatillon_Centrale/RConn3 -- bus686/LConn1
  T_103007085_220000_Montjovet_centrale/RConn1 -- L_103007085/LConn1
  T_103007085_220000_Montjovet_centrale/RConn2 -- L_103007085/LConn2
  L_103007085/LConn3 -- T_103007085_220000_Montjovet_centrale/RConn3 -- bus687/LConn1
  T_105153431_380000_Leinì/RConn1 -- L_105153431/LConn1
  T_105153431_380000_Leinì/RConn2 -- L_105153431/LConn2
  L_105153431/LConn3 -- T_105153431_380000_Leinì/RConn3 -- bus688/LConn1
  T_103127417_220000_Valpelline_G2/RConn1 -- L_103127417/LConn1
  T_103127417_220000_Valpelline_G2/RConn2 -- L_103127417/LConn2
  L_103127417/LConn3 -- T_103127417_220000_Valpelline_G2/RConn3 -- bus689/LConn1
  T_189137043_220000_Gargnano/RConn1 -- L_189137043/LConn1
  T_189137043_220000_Gargnano/RConn2 -- L_189137043/LConn2
  L_189137043/LConn3 -- T_189137043_220000_Gargnano/RConn3 -- bus690/LConn1
  T_320030656_220000_Tecnoparco/RConn1 -- L_320030656/LConn1
  T_320030656_220000_Tecnoparco/RConn2 -- L_320030656/LConn2
  L_320030656/LConn3 -- T_320030656_220000_Tecnoparco/RConn3 -- bus691/LConn1
  T_348500306_220000_Campo_Moro/RConn1 -- L_348500306/LConn1
  T_348500306_220000_Campo_Moro/RConn2 -- L_348500306/LConn2
  L_348500306/LConn3 -- T_348500306_220000_Campo_Moro/RConn3 -- bus692/LConn1
  T_105581403_380000_Chivasso_Termica_380kV/RConn1 -- L_105581403/LConn1
  T_105581403_380000_Chivasso_Termica_380kV/RConn2 -- L_105581403/LConn2
  L_105581403/LConn3 -- T_105581403_380000_Chivasso_Termica_380kV/RConn3 -- bus693/LConn1
  T_102287716_220000_Chivasso_Termica_220kV/RConn1 -- L_102287716/LConn1
  T_102287716_220000_Chivasso_Termica_220kV/RConn2 -- L_102287716/LConn2
  L_102287716/LConn3 -- T_102287716_220000_Chivasso_Termica_220kV/RConn3 -- bus694/LConn1
  T_57403755_220000_Ciminna/RConn1 -- L_57403755/LConn1
  T_57403755_220000_Ciminna/RConn2 -- L_57403755/LConn2
  L_57403755/LConn3 -- T_57403755_220000_Ciminna/RConn3 -- bus695/LConn1
  T_207383904_220000_Arenella/RConn1 -- L_207383904/LConn1
  T_207383904_220000_Arenella/RConn2 -- L_207383904/LConn2
  L_207383904/LConn3 -- T_207383904_220000_Arenella/RConn3 -- bus696/LConn1
  T_377588144_220000_/RConn1 -- L_377588144/LConn1
  T_377588144_220000_/RConn2 -- L_377588144/LConn2
  L_377588144/LConn3 -- T_377588144_220000_/RConn3 -- bus697/LConn1
  T_149071351_220000_Acciaieria_Valsugana/RConn1 -- L_149071351/LConn1
  T_149071351_220000_Acciaieria_Valsugana/RConn2 -- L_149071351/LConn2
  L_149071351/LConn3 -- T_149071351_220000_Acciaieria_Valsugana/RConn3 -- bus698/LConn1
  T_147453809_220000_Santa_Massenza_sezione_220K/RConn1 -- L_147453809/LConn1
  T_147453809_220000_Santa_Massenza_sezione_220K/RConn2 -- L_147453809/LConn2
  L_147453809/LConn3 -- T_147453809_220000_Santa_Massenza_sezione_220K/RConn3 -- bus699/LConn1
  T_107683818_380000_Stazione_elettrica_Marginone/RConn1 -- L_107683818/LConn1
  T_107683818_380000_Stazione_elettrica_Marginone/RConn2 -- L_107683818/LConn2
  L_107683818/LConn3 -- T_107683818_380000_Stazione_elettrica_Marginone/RConn3 -- bus700/LConn1
  T_107843509_220000_Livorno_Marzocco/RConn1 -- L_107843509/LConn1
  T_107843509_220000_Livorno_Marzocco/RConn2 -- L_107843509/LConn2
  L_107843509/LConn3 -- T_107843509_220000_Livorno_Marzocco/RConn3 -- bus701/LConn1
  T_375922075_220000_Eni_Versalis/RConn1 -- L_375922075/LConn1
  T_375922075_220000_Eni_Versalis/RConn2 -- L_375922075/LConn2
  L_375922075/LConn3 -- T_375922075_220000_Eni_Versalis/RConn3 -- bus702/LConn1
  T_60919237_380000_Brindisi/RConn1 -- L_60919237/LConn1
  T_60919237_380000_Brindisi/RConn2 -- L_60919237/LConn2
  L_60919237/LConn3 -- T_60919237_380000_Brindisi/RConn3 -- bus703/LConn1
  T_377438327_220000_Imi_sud/RConn1 -- L_377438327/LConn1
  T_377438327_220000_Imi_sud/RConn2 -- L_377438327/LConn2
  L_377438327/LConn3 -- T_377438327_220000_Imi_sud/RConn3 -- bus704/LConn1
  T_82793962_220000_Cimego/RConn1 -- L_82793962/LConn1
  T_82793962_220000_Cimego/RConn2 -- L_82793962/LConn2
  L_82793962/LConn3 -- T_82793962_220000_Cimego/RConn3 -- bus705/LConn1
  T_339706880_380000_Tuscania/RConn1 -- L_339706880/LConn1
  T_339706880_380000_Tuscania/RConn2 -- L_339706880/LConn2
  L_339706880/LConn3 -- T_339706880_380000_Tuscania/RConn3 -- bus706/LConn1
  T_59219335_380000_Montalto/RConn1 -- L_59219335/LConn1
  T_59219335_380000_Montalto/RConn2 -- L_59219335/LConn2
  L_59219335/LConn3 -- T_59219335_380000_Montalto/RConn3 -- bus707/LConn1
  T_339706881_380000_Villavalle/RConn1 -- L_339706881/LConn1
  T_339706881_380000_Villavalle/RConn2 -- L_339706881/LConn2
  L_339706881/LConn3 -- T_339706881_380000_Villavalle/RConn3 -- bus708/LConn1
  T_60913666_380000_Bari_Ovest/RConn1 -- L_60913666/LConn1
  T_60913666_380000_Bari_Ovest/RConn2 -- L_60913666/LConn2
  L_60913666/LConn3 -- T_60913666_380000_Bari_Ovest/RConn3 -- bus709/LConn1
  T_146791061_380000_Palo_del_Colle/RConn1 -- L_146791061/LConn1
  T_146791061_380000_Palo_del_Colle/RConn2 -- L_146791061/LConn2
  L_146791061/LConn3 -- T_146791061_380000_Palo_del_Colle/RConn3 -- bus710/LConn1
  T_416989699_380000_Montalto_centrale/RConn1 -- L_416989699/LConn1
  T_416989699_380000_Montalto_centrale/RConn2 -- L_416989699/LConn2
  L_416989699/LConn3 -- T_416989699_380000_Montalto_centrale/RConn3 -- bus711/LConn1
  T_114931087_380000_Bargi/RConn1 -- L_114931087/LConn1
  T_114931087_380000_Bargi/RConn2 -- L_114931087/LConn2
  L_114931087/LConn3 -- T_114931087_380000_Bargi/RConn3 -- bus712/LConn1
  T_72570378_380000_Musignano/RConn1 -- L_72570378/LConn1
  T_72570378_380000_Musignano/RConn2 -- L_72570378/LConn2
  L_72570378/LConn3 -- T_72570378_380000_Musignano/RConn3 -- bus713/LConn1
  T_72581705_380000_Mercallo/RConn1 -- L_72581705/LConn1
  T_72581705_380000_Mercallo/RConn2 -- L_72581705/LConn2
  L_72581705/LConn3 -- T_72581705_380000_Mercallo/RConn3 -- bus714/LConn1
  T_75604825_380000_Roncovalgrande/RConn1 -- L_75604825/LConn1
  T_75604825_380000_Roncovalgrande/RConn2 -- L_75604825/LConn2
  L_75604825/LConn3 -- T_75604825_380000_Roncovalgrande/RConn3 -- bus715/LConn1
  T_72570474_380000_Cagno/RConn1 -- L_72570474/LConn1
  T_72570474_380000_Cagno/RConn2 -- L_72570474/LConn2
  L_72570474/LConn3 -- T_72570474_380000_Cagno/RConn3 -- bus716/LConn1
  T_39255054_380000_Parma_Vigheffio/RConn1 -- L_39255054/LConn1
  T_39255054_380000_Parma_Vigheffio/RConn2 -- L_39255054/LConn2
  L_39255054/LConn3 -- T_39255054_380000_Parma_Vigheffio/RConn3 -- bus717/LConn1
  T_78066534_380000_Rubiera/RConn1 -- L_78066534/LConn1
  T_78066534_380000_Rubiera/RConn2 -- L_78066534/LConn2
  L_78066534/LConn3 -- T_78066534_380000_Rubiera/RConn3 -- bus718/LConn1
  T_93315059_380000_San_Rocco_Po/RConn1 -- L_93315059/LConn1
  T_93315059_380000_San_Rocco_Po/RConn2 -- L_93315059/LConn2
  L_93315059/LConn3 -- T_93315059_380000_San_Rocco_Po/RConn3 -- bus719/LConn1
  T_105757794_380000_La_Spezia/RConn1 -- L_105757794/LConn1
  T_105757794_380000_La_Spezia/RConn2 -- L_105757794/LConn2
  L_105757794/LConn3 -- T_105757794_380000_La_Spezia/RConn3 -- bus720/LConn1
  T_303965869_380000_Maida/RConn1 -- L_303965869/LConn1
  T_303965869_380000_Maida/RConn2 -- L_303965869/LConn2
  L_303965869/LConn3 -- T_303965869_380000_Maida/RConn3 -- bus721/LConn1
  T_109993642_380000_Rizziconi/RConn1 -- L_109993642/LConn1
  T_109993642_380000_Rizziconi/RConn2 -- L_109993642/LConn2
  L_109993642/LConn3 -- T_109993642_380000_Rizziconi/RConn3 -- bus722/LConn1
  T_199676823_380000_Magisano/RConn1 -- L_199676823/LConn1
  T_199676823_380000_Magisano/RConn2 -- L_199676823/LConn2
  L_199676823/LConn3 -- T_199676823_380000_Magisano/RConn3 -- bus723/LConn1
  T_98421779_380000_Trino_Centrale/RConn1 -- L_98421779/LConn1
  T_98421779_380000_Trino_Centrale/RConn2 -- L_98421779/LConn2
  L_98421779/LConn3 -- T_98421779_380000_Trino_Centrale/RConn3 -- bus724/LConn1
  T_98427149_380000_Castelnuovo/RConn1 -- L_98427149/LConn1
  T_98427149_380000_Castelnuovo/RConn2 -- L_98427149/LConn2
  L_98427149/LConn3 -- T_98427149_380000_Castelnuovo/RConn3 -- bus725/LConn1
  T_236661269_380000_Lacchiarella/RConn1 -- L_236661269/LConn1
  T_236661269_380000_Lacchiarella/RConn2 -- L_236661269/LConn2
  L_236661269/LConn3 -- T_236661269_380000_Lacchiarella/RConn3 -- bus726/LConn1
  T_202271565_380000_Chignolo_Po/RConn1 -- L_202271565/LConn1
  T_202271565_380000_Chignolo_Po/RConn2 -- L_202271565/LConn2
  L_202271565/LConn3 -- T_202271565_380000_Chignolo_Po/RConn3 -- bus727/LConn1
  T_338760116_380000_Castellaneta/RConn1 -- L_338760116/LConn1
  T_338760116_380000_Castellaneta/RConn2 -- L_338760116/LConn2
  L_338760116/LConn3 -- T_338760116_380000_Castellaneta/RConn3 -- bus728/LConn1
  T_103386958_380000_Galatina/RConn1 -- L_103386958/LConn1
  T_103386958_380000_Galatina/RConn2 -- L_103386958/LConn2
  L_103386958/LConn3 -- T_103386958_380000_Galatina/RConn3 -- bus729/LConn1
  T_82084019_380000_Sermide/RConn1 -- L_82084019/LConn1
  T_82084019_380000_Sermide/RConn2 -- L_82084019/LConn2
  L_82084019/LConn3 -- T_82084019_380000_Sermide/RConn3 -- bus730/LConn1
  T_82084013_380000_Ferrara_Nord/RConn1 -- L_82084013/LConn1
  T_82084013_380000_Ferrara_Nord/RConn2 -- L_82084013/LConn2
  L_82084013/LConn3 -- T_82084013_380000_Ferrara_Nord/RConn3 -- bus731/LConn1
  T_421827452_380000_Ostiglia_centrale/RConn1 -- L_421827452/LConn1
  T_421827452_380000_Ostiglia_centrale/RConn2 -- L_421827452/LConn2
  L_421827452/LConn3 -- T_421827452_380000_Ostiglia_centrale/RConn3 -- bus732/LConn1
  T_116697005_380000_Mantova/RConn1 -- L_116697005/LConn1
  T_116697005_380000_Mantova/RConn2 -- L_116697005/LConn2
  L_116697005/LConn3 -- T_116697005_380000_Mantova/RConn3 -- bus733/LConn1
  T_149997403_380000_Eni_Power/RConn1 -- L_149997403/LConn1
  T_149997403_380000_Eni_Power/RConn2 -- L_149997403/LConn2
  L_149997403/LConn3 -- T_149997403_380000_Eni_Power/RConn3 -- bus734/LConn1
  "T_81938081_380000_Stazione_elettrica_\"Ravenna_Canala\""/RConn1 -- L_81938081/LConn1
  "T_81938081_380000_Stazione_elettrica_\"Ravenna_Canala\""/RConn2 -- L_81938081/LConn2
  L_81938081/LConn3 -- "T_81938081_380000_Stazione_elettrica_\"Ravenna_Canala\""/RConn3 -- bus735/LConn1
  T_75947556_380000_Ciserano/RConn1 -- L_75947556/LConn1
  T_75947556_380000_Ciserano/RConn2 -- L_75947556/LConn2
  L_75947556/LConn3 -- T_75947556_380000_Ciserano/RConn3 -- bus736/LConn1
  T_133601335_380000_Cassano/RConn1 -- L_133601335/LConn1
  T_133601335_380000_Cassano/RConn2 -- L_133601335/LConn2
  L_133601335/LConn3 -- T_133601335_380000_Cassano/RConn3 -- bus737/LConn1
  T_60725875_380000_Monfalcone_sezione_1_400/RConn1 -- L_60725875/LConn1
  T_60725875_380000_Monfalcone_sezione_1_400/RConn2 -- L_60725875/LConn2
  L_60725875/LConn3 -- T_60725875_380000_Monfalcone_sezione_1_400/RConn3 -- bus738/LConn1
  T_58992998_380000_Planais/RConn1 -- L_58992998/LConn1
  T_58992998_380000_Planais/RConn2 -- L_58992998/LConn2
  L_58992998/LConn3 -- T_58992998_380000_Planais/RConn3 -- bus739/LConn1
  T_61626687_380000_Teramo/RConn1 -- L_61626687/LConn1
  T_61626687_380000_Teramo/RConn2 -- L_61626687/LConn2
  L_61626687/LConn3 -- T_61626687_380000_Teramo/RConn3 -- bus740/LConn1
  T_74943205_380000_Fano_Entroterra/RConn1 -- L_74943205/LConn1
  T_74943205_380000_Fano_Entroterra/RConn2 -- L_74943205/LConn2
  L_74943205/LConn3 -- T_74943205_380000_Fano_Entroterra/RConn3 -- bus741/LConn1
  T_110330925_380000_Altomonte_Centrale/RConn1 -- L_110330925/LConn1
  T_110330925_380000_Altomonte_Centrale/RConn2 -- L_110330925/LConn2
  L_110330925/LConn3 -- T_110330925_380000_Altomonte_Centrale/RConn3 -- bus742/LConn1
  T_110310021_380000_Stazione_Elettrica_di_Feroleto/RConn1 -- L_110310021/LConn1
  T_110310021_380000_Stazione_Elettrica_di_Feroleto/RConn2 -- L_110310021/LConn2
  L_110310021/LConn3 -- T_110310021_380000_Stazione_Elettrica_di_Feroleto/RConn3 -- bus743/LConn1
  T_338792752_380000_San_Severo/RConn1 -- L_338792752/LConn1
  T_338792752_380000_San_Severo/RConn2 -- L_338792752/LConn2
  L_338792752/LConn3 -- T_338792752_380000_San_Severo/RConn3 -- bus744/LConn1
  T_418565264_380000_Ratino_centrale/RConn1 -- L_418565264/LConn1
  T_418565264_380000_Ratino_centrale/RConn2 -- L_418565264/LConn2
  L_418565264/LConn3 -- T_418565264_380000_Ratino_centrale/RConn3 -- bus745/LConn1
  T_60235685_380000_Larino/RConn1 -- L_60235685/LConn1
  T_60235685_380000_Larino/RConn2 -- L_60235685/LConn2
  L_60235685/LConn3 -- T_60235685_380000_Larino/RConn3 -- bus746/LConn1
  T_418565263_380000_Foggia/RConn1 -- L_418565263/LConn1
  T_418565263_380000_Foggia/RConn2 -- L_418565263/LConn2
  L_418565263/LConn3 -- T_418565263_380000_Foggia/RConn3 -- bus747/LConn1
  T_107681459_380000_Acciaiolo/RConn1 -- L_107681459/LConn1
  T_107681459_380000_Acciaiolo/RConn2 -- L_107681459/LConn2
  L_107681459/LConn3 -- T_107681459_380000_Acciaiolo/RConn3 -- bus748/LConn1
  T_116240715_380000_Roselectra/RConn1 -- L_116240715/LConn1
  T_116240715_380000_Roselectra/RConn2 -- L_116240715/LConn2
  L_116240715/LConn3 -- T_116240715_380000_Roselectra/RConn3 -- bus749/LConn1
  T_157912118_380000_Stazione_Elettrica_Paradiso/RConn1 -- L_157912118/LConn1
  T_157912118_380000_Stazione_Elettrica_Paradiso/RConn2 -- L_157912118/LConn2
  L_157912118/LConn3 -- T_157912118_380000_Stazione_Elettrica_Paradiso/RConn3 -- bus750/LConn1
  T_109997676_380000_Bolano/RConn1 -- L_109997676/LConn1
  T_109997676_380000_Bolano/RConn2 -- L_109997676/LConn2
  L_109997676/LConn3 -- T_109997676_380000_Bolano/RConn3 -- bus751/LConn1
  T_59462715_380000_Torviscosa_Edison/RConn1 -- L_59462715/LConn1
  T_59462715_380000_Torviscosa_Edison/RConn2 -- L_59462715/LConn2
  L_59462715/LConn3 -- T_59462715_380000_Torviscosa_Edison/RConn3 -- bus752/LConn1
  T_199675964_380000_Simeri_Crichi/RConn1 -- L_199675964/LConn1
  T_199675964_380000_Simeri_Crichi/RConn2 -- L_199675964/LConn2
  L_199675964/LConn3 -- T_199675964_380000_Simeri_Crichi/RConn3 -- bus753/LConn1
  T_189612607_380000_Rho/RConn1 -- L_189612607/LConn1
  T_189612607_380000_Rho/RConn2 -- L_189612607/LConn2
  L_189612607/LConn3 -- T_189612607_380000_Rho/RConn3 -- bus754/LConn1
  T_74677138_380000_Bovisio/RConn1 -- L_74677138/LConn1
  T_74677138_380000_Bovisio/RConn2 -- L_74677138/LConn2
  L_74677138/LConn3 -- T_74677138_380000_Bovisio/RConn3 -- bus755/LConn1
  T_34157795_380000_Ospiate/RConn1 -- L_34157795/LConn1
  T_34157795_380000_Ospiate/RConn2 -- L_34157795/LConn2
  L_34157795/LConn3 -- T_34157795_380000_Ospiate/RConn3 -- bus756/LConn1
  T_93038661_380000_Pieve_Albignola/RConn1 -- L_93038661/LConn1
  T_93038661_380000_Pieve_Albignola/RConn2 -- L_93038661/LConn2
  L_93038661/LConn3 -- T_93038661_380000_Pieve_Albignola/RConn3 -- bus757/LConn1
  T_98901130_380000_Voghera/RConn1 -- L_98901130/LConn1
  T_98901130_380000_Voghera/RConn2 -- L_98901130/LConn2
  L_98901130/LConn3 -- T_98901130_380000_Voghera/RConn3 -- bus758/LConn1
  T_208398923_380000_Carpi_Fossoli/RConn1 -- L_208398923/LConn1
  T_208398923_380000_Carpi_Fossoli/RConn2 -- L_208398923/LConn2
  L_208398923/LConn3 -- T_208398923_380000_Carpi_Fossoli/RConn3 -- bus759/LConn1
  T_148969091_380000;132000;15000_San_Damaso/RConn1 -- L_148969091/LConn1
  T_148969091_380000;132000;15000_San_Damaso/RConn2 -- L_148969091/LConn2
  L_148969091/LConn3 -- T_148969091_380000;132000;15000_San_Damaso/RConn3 -- bus760/LConn1
  T_116517585_380000_Caorso/RConn1 -- L_116517585/LConn1
  T_116517585_380000_Caorso/RConn2 -- L_116517585/LConn2
  L_116517585/LConn3 -- T_116517585_380000_Caorso/RConn3 -- bus761/LConn1
  T_83805453_380000_Pian_della_Speranza/RConn1 -- L_83805453/LConn1
  T_83805453_380000_Pian_della_Speranza/RConn2 -- L_83805453/LConn2
  L_83805453/LConn3 -- T_83805453_380000_Pian_della_Speranza/RConn3 -- bus762/LConn1
  T_58931857_380000_Valmontone/RConn1 -- L_58931857/LConn1
  T_58931857_380000_Valmontone/RConn2 -- L_58931857/LConn2
  L_58931857/LConn3 -- T_58931857_380000_Valmontone/RConn3 -- bus763/LConn1
  T_84301904_380000_Venezia_Nord/RConn1 -- L_84301904/LConn1
  T_84301904_380000_Venezia_Nord/RConn2 -- L_84301904/LConn2
  L_84301904/LConn3 -- T_84301904_380000_Venezia_Nord/RConn3 -- bus764/LConn1
  T_109756016_380000_Scandale/RConn1 -- L_109756016/LConn1
  T_109756016_380000_Scandale/RConn2 -- L_109756016/LConn2
  L_109756016/LConn3 -- T_109756016_380000_Scandale/RConn3 -- bus765/LConn1
  T_418902799_380000_Brindisi_Sud_centrale_GR_1/RConn1 -- L_418902799/LConn1
  T_418902799_380000_Brindisi_Sud_centrale_GR_1/RConn2 -- L_418902799/LConn2
  L_418902799/LConn3 -- T_418902799_380000_Brindisi_Sud_centrale_GR_1/RConn3 -- bus766/LConn1
  T_60888331_380000_Brindisi_Sud/RConn1 -- L_60888331/LConn1
  T_60888331_380000_Brindisi_Sud/RConn2 -- L_60888331/LConn2
  L_60888331/LConn3 -- T_60888331_380000_Brindisi_Sud/RConn3 -- bus767/LConn1
  T_140710344_380000_Tavarnuzze/RConn1 -- L_140710344/LConn1
  T_140710344_380000_Tavarnuzze/RConn2 -- L_140710344/LConn2
  L_140710344/LConn3 -- T_140710344_380000_Tavarnuzze/RConn3 -- bus768/LConn1
  T_363469921_380000_Stazione_elettrica_di_Focomorto/RConn1 -- L_363469921/LConn1
  T_363469921_380000_Stazione_elettrica_di_Focomorto/RConn2 -- L_363469921/LConn2
  L_363469921/LConn3 -- T_363469921_380000_Stazione_elettrica_di_Focomorto/RConn3 -- bus769/LConn1
  T_59462263_380000_Udine_Ovest/RConn1 -- L_59462263/LConn1
  T_59462263_380000_Udine_Ovest/RConn2 -- L_59462263/LConn2
  L_59462263/LConn3 -- T_59462263_380000_Udine_Ovest/RConn3 -- bus770/LConn1
  T_109588422_380000_Rossano_Termica/RConn1 -- L_109588422/LConn1
  T_109588422_380000_Rossano_Termica/RConn2 -- L_109588422/LConn2
  L_109588422/LConn3 -- T_109588422_380000_Rossano_Termica/RConn3 -- bus771/LConn1
  T_82083756_380000_Cordignano/RConn1 -- L_82083756/LConn1
  T_82083756_380000_Cordignano/RConn2 -- L_82083756/LConn2
  L_82083756/LConn3 -- T_82083756_380000_Cordignano/RConn3 -- bus772/LConn1
  T_338453112_380000_Martignone/RConn1 -- L_338453112/LConn1
  T_338453112_380000_Martignone/RConn2 -- L_338453112/LConn2
  L_338453112/LConn3 -- T_338453112_380000_Martignone/RConn3 -- bus773/LConn1
  T_81931074_380000_Forlì_via_Oraziana/RConn1 -- L_81931074/LConn1
  T_81931074_380000_Forlì_via_Oraziana/RConn2 -- L_81931074/LConn2
  L_81931074/LConn3 -- T_81931074_380000_Forlì_via_Oraziana/RConn3 -- bus774/LConn1
  T_95840602_380000_RFX/RConn1 -- L_95840602/LConn1
  T_95840602_380000_RFX/RConn2 -- L_95840602/LConn2
  L_95840602/LConn3 -- T_95840602_380000_RFX/RConn3 -- bus775/LConn1
  T_146652797_380000_/RConn1 -- L_146652797/LConn1
  T_146652797_380000_/RConn2 -- L_146652797/LConn2
  L_146652797/LConn3 -- T_146652797_380000_/RConn3 -- bus776/LConn1
  T_152597636_380000_Bulciago/RConn1 -- L_152597636/LConn1
  T_152597636_380000_Bulciago/RConn2 -- L_152597636/LConn2
  L_152597636/LConn3 -- T_152597636_380000_Bulciago/RConn3 -- bus777/LConn1
  T_60616350_380000_Gissi_Centrale/RConn1 -- L_60616350/LConn1
  T_60616350_380000_Gissi_Centrale/RConn2 -- L_60616350/LConn2
  L_60616350/LConn3 -- T_60616350_380000_Gissi_Centrale/RConn3 -- bus778/LConn1
  T_411026199_380000_ENM_Termoli/RConn1 -- L_411026199/LConn1
  T_411026199_380000_ENM_Termoli/RConn2 -- L_411026199/LConn2
  L_411026199/LConn3 -- T_411026199_380000_ENM_Termoli/RConn3 -- bus779/LConn1
  T_131291789_380000_Lonato/RConn1 -- L_131291789/LConn1
  T_131291789_380000_Lonato/RConn2 -- L_131291789/LConn2
  L_131291789/LConn3 -- T_131291789_380000_Lonato/RConn3 -- bus780/LConn1
  T_155791516_380000_Nogarole_Rocca/RConn1 -- L_155791516/LConn1
  T_155791516_380000_Nogarole_Rocca/RConn2 -- L_155791516/LConn2
  L_155791516/LConn3 -- T_155791516_380000_Nogarole_Rocca/RConn3 -- bus781/LConn1
  T_209982720_380000_Troia/RConn1 -- L_209982720/LConn1
  T_209982720_380000_Troia/RConn2 -- L_209982720/LConn2
  L_209982720/LConn3 -- T_209982720_380000_Troia/RConn3 -- bus782/LConn1
  T_338795626_380000_Deliceto/RConn1 -- L_338795626/LConn1
  T_338795626_380000_Deliceto/RConn2 -- L_338795626/LConn2
  L_338795626/LConn3 -- T_338795626_380000_Deliceto/RConn3 -- bus783/LConn1
  T_126203383_380000_Andria/RConn1 -- L_126203383/LConn1
  T_126203383_380000_Andria/RConn2 -- L_126203383/LConn2
  L_126203383/LConn3 -- T_126203383_380000_Andria/RConn3 -- bus784/LConn1
  T_82921983_380000_Presenzano/RConn1 -- L_82921983/LConn1
  T_82921983_380000_Presenzano/RConn2 -- L_82921983/LConn2
  L_82921983/LConn3 -- T_82921983_380000_Presenzano/RConn3 -- bus785/LConn1
  T_76709660_380000_Roma_Est/RConn1 -- L_76709660/LConn1
  T_76709660_380000_Roma_Est/RConn2 -- L_76709660/LConn2
  L_76709660/LConn3 -- T_76709660_380000_Roma_Est/RConn3 -- bus786/LConn1
  T_339704025_380000_Latina/RConn1 -- L_339704025/LConn1
  T_339704025_380000_Latina/RConn2 -- L_339704025/LConn2
  L_339704025/LConn3 -- T_339704025_380000_Latina/RConn3 -- bus787/LConn1
  T_104359058_380000_Entracque/RConn1 -- L_104359058/LConn1
  T_104359058_380000_Entracque/RConn2 -- L_104359058/LConn2
  L_104359058/LConn3 -- T_104359058_380000_Entracque/RConn3 -- bus788/LConn1
  T_99694910_380000_Magliano/RConn1 -- L_99694910/LConn1
  T_99694910_380000_Magliano/RConn2 -- L_99694910/LConn2
  L_99694910/LConn3 -- T_99694910_380000_Magliano/RConn3 -- bus789/LConn1
  T_338753171_380000_Priolo/RConn1 -- L_338753171/LConn1
  T_338753171_380000_Priolo/RConn2 -- L_338753171/LConn2
  L_338753171/LConn3 -- T_338753171_380000_Priolo/RConn3 -- bus790/LConn1
  T_415431845_380000_Isab_Energy/RConn1 -- L_415431845/LConn1
  T_415431845_380000_Isab_Energy/RConn2 -- L_415431845/LConn2
  L_415431845/LConn3 -- T_415431845_380000_Isab_Energy/RConn3 -- bus791/LConn1
  T_146791215__/RConn1 -- L_146791215/LConn1
  T_146791215__/RConn2 -- L_146791215/LConn2
  L_146791215/LConn3 -- T_146791215__/RConn3 -- bus792/LConn1
  T_171270810_380000_Candela/RConn1 -- L_171270810/LConn1
  T_171270810_380000_Candela/RConn2 -- L_171270810/LConn2
  L_171270810/LConn3 -- T_171270810_380000_Candela/RConn3 -- bus793/LConn1
  T_81929591_380000_Porto_Tolle/RConn1 -- L_81929591/LConn1
  T_81929591_380000_Porto_Tolle/RConn2 -- L_81929591/LConn2
  L_81929591/LConn3 -- T_81929591_380000_Porto_Tolle/RConn3 -- bus794/LConn1
  T_158739183_380000_Porto_Corsini_Sezione_1/RConn1 -- L_158739183/LConn1
  T_158739183_380000_Porto_Corsini_Sezione_1/RConn2 -- L_158739183/LConn2
  L_158739183/LConn3 -- T_158739183_380000_Porto_Corsini_Sezione_1/RConn3 -- bus795/LConn1
  T_64200868_380000_Stazione_Primaria_di_Edolo/RConn1 -- L_64200868/LConn1
  T_64200868_380000_Stazione_Primaria_di_Edolo/RConn2 -- L_64200868/LConn2
  L_64200868/LConn3 -- T_64200868_380000_Stazione_Primaria_di_Edolo/RConn3 -- bus796/LConn1
  T_72466334_380000_San_Fiorano/RConn1 -- L_72466334/LConn1
  T_72466334_380000_San_Fiorano/RConn2 -- L_72466334/LConn2
  L_72466334/LConn3 -- T_72466334_380000_San_Fiorano/RConn3 -- bus797/LConn1
  T_365525159_380000_SEF_Ferrara/RConn1 -- L_365525159/LConn1
  T_365525159_380000_SEF_Ferrara/RConn2 -- L_365525159/LConn2
  L_365525159/LConn3 -- T_365525159_380000_SEF_Ferrara/RConn3 -- bus798/LConn1
  T_103306951_380000_Matera/RConn1 -- L_103306951/LConn1
  T_103306951_380000_Matera/RConn2 -- L_103306951/LConn2
  L_103306951/LConn3 -- T_103306951_380000_Matera/RConn3 -- bus799/LConn1
  T_338790588_380000_Aliano/RConn1 -- L_338790588/LConn1
  T_338790588_380000_Aliano/RConn2 -- L_338790588/LConn2
  L_338790588/LConn3 -- T_338790588_380000_Aliano/RConn3 -- bus800/LConn1
  T_257351439_380000_Bisaccia_380/RConn1 -- L_257351439/LConn1
  T_257351439_380000_Bisaccia_380/RConn2 -- L_257351439/LConn2
  L_257351439/LConn3 -- T_257351439_380000_Bisaccia_380/RConn3 -- bus801/LConn1
  T_409439916_380000_Fiumesanto_Carbo_380/RConn1 -- L_409439916/LConn1
  T_409439916_380000_Fiumesanto_Carbo_380/RConn2 -- L_409439916/LConn2
  L_409439916/LConn3 -- T_409439916_380000_Fiumesanto_Carbo_380/RConn3 -- bus802/LConn1
  T_144005863_380000_Ittiri/RConn1 -- L_144005863/LConn1
  T_144005863_380000_Ittiri/RConn2 -- L_144005863/LConn2
  L_144005863/LConn3 -- T_144005863_380000_Ittiri/RConn3 -- bus803/LConn1
  T_140715391_380000_Le_Rose/RConn1 -- L_140715391/LConn1
  T_140715391_380000_Le_Rose/RConn2 -- L_140715391/LConn2
  L_140715391/LConn3 -- T_140715391_380000_Le_Rose/RConn3 -- bus804/LConn1
  T_58440884_380000_Flero/RConn1 -- L_58440884/LConn1
  T_58440884_380000_Flero/RConn2 -- L_58440884/LConn2
  L_58440884/LConn3 -- T_58440884_380000_Flero/RConn3 -- bus805/LConn1
  T_211180338_380000_Maleo/RConn1 -- L_211180338/LConn1
  T_211180338_380000_Maleo/RConn2 -- L_211180338/LConn2
  L_211180338/LConn3 -- T_211180338_380000_Maleo/RConn3 -- bus806/LConn1
  T_116518388_380000_Cremona/RConn1 -- L_116518388/LConn1
  T_116518388_380000_Cremona/RConn2 -- L_116518388/LConn2
  L_116518388/LConn3 -- T_116518388_380000_Cremona/RConn3 -- bus807/LConn1
  T_120356593_380000_Travagliato/RConn1 -- L_120356593/LConn1
  T_120356593_380000_Travagliato/RConn2 -- L_120356593/LConn2
  L_120356593/LConn3 -- T_120356593_380000_Travagliato/RConn3 -- bus808/LConn1
  T_64942789_380000;132000_Sandrigo/RConn1 -- L_64942789/LConn1
  T_64942789_380000;132000_Sandrigo/RConn2 -- L_64942789/LConn2
  L_64942789/LConn3 -- T_64942789_380000;132000_Sandrigo/RConn3 -- bus809/LConn1
  T_158086858__/RConn1 -- L_158086858/LConn1
  T_158086858__/RConn2 -- L_158086858/LConn2
  L_158086858/LConn3 -- T_158086858__/RConn3 -- bus810/LConn1
  T_158183759__/RConn1 -- L_158183759/LConn1
  T_158183759__/RConn2 -- L_158183759/LConn2
  L_158183759/LConn3 -- T_158183759__/RConn3 -- bus811/LConn1
  T_339703159_380000_Santa_Barbara/RConn1 -- L_339703159/LConn1
  T_339703159_380000_Santa_Barbara/RConn2 -- L_339703159/LConn2
  L_339703159/LConn3 -- T_339703159_380000_Santa_Barbara/RConn3 -- bus812/LConn1
  T_83872215_380000_Garigliano/RConn1 -- L_83872215/LConn1
  T_83872215_380000_Garigliano/RConn2 -- L_83872215/LConn2
  L_83872215/LConn3 -- T_83872215_380000_Garigliano/RConn3 -- bus813/LConn1
  T_82759380_380000_Aurelia/RConn1 -- L_82759380/LConn1
  T_82759380_380000_Aurelia/RConn2 -- L_82759380/LConn2
  L_82759380/LConn3 -- T_82759380_380000_Aurelia/RConn3 -- bus814/LConn1
  T_82114903_380000_Torrevaldiga_Nord/RConn1 -- L_82114903/LConn1
  T_82114903_380000_Torrevaldiga_Nord/RConn2 -- L_82114903/LConn2
  L_82114903/LConn3 -- T_82114903_380000_Torrevaldiga_Nord/RConn3 -- bus815/LConn1
  T_103653592_380000_Vado_Termica/RConn1 -- L_103653592/LConn1
  T_103653592_380000_Vado_Termica/RConn2 -- L_103653592/LConn2
  L_103653592/LConn3 -- T_103653592_380000_Vado_Termica/RConn3 -- bus816/LConn1
  T_83058212_380000_Benevento_2/RConn1 -- L_83058212/LConn1
  T_83058212_380000_Benevento_2/RConn2 -- L_83058212/LConn2
  L_83058212/LConn3 -- T_83058212_380000_Benevento_2/RConn3 -- bus817/LConn1
  T_116797658_380000_Mantova_380/RConn1 -- L_116797658/LConn1
  T_116797658_380000_Mantova_380/RConn2 -- L_116797658/LConn2
  L_116797658/LConn3 -- T_116797658_380000_Mantova_380/RConn3 -- bus818/LConn1
  T_116912085__/RConn1 -- L_116912085/LConn1
  T_116912085__/RConn2 -- L_116912085/LConn2
  L_116912085/LConn3 -- T_116912085__/RConn3 -- bus819/LConn1
  T_255011550_380000_Sarlux/RConn1 -- L_255011550/LConn1
  T_255011550_380000_Sarlux/RConn2 -- L_255011550/LConn2
  L_255011550/LConn3 -- T_255011550_380000_Sarlux/RConn3 -- bus820/LConn1
  T_255011551_380000_Cagliari_Sud/RConn1 -- L_255011551/LConn1
  T_255011551_380000_Cagliari_Sud/RConn2 -- L_255011551/LConn2
  L_255011551/LConn3 -- T_255011551_380000_Cagliari_Sud/RConn3 -- bus821/LConn1
  T_74210017__Pogliano/RConn1 -- L_74210017/LConn1
  T_74210017__Pogliano/RConn2 -- L_74210017/LConn2
  L_74210017/LConn3 -- T_74210017__Pogliano/RConn3 -- bus822/LConn1
  T_143585004_380000_San_Martino_in_XX/RConn1 -- L_143585004/LConn1
  T_143585004_380000_San_Martino_in_XX/RConn2 -- L_143585004/LConn2
  L_143585004/LConn3 -- T_143585004_380000_San_Martino_in_XX/RConn3 -- bus823/LConn1
  T_98900549_380000_Ferrera_Erbognone/RConn1 -- L_98900549/LConn1
  T_98900549_380000_Ferrera_Erbognone/RConn2 -- L_98900549/LConn2
  L_98900549/LConn3 -- T_98900549_380000_Ferrera_Erbognone/RConn3 -- bus824/LConn1
  T_72475426_380000_Chiari/RConn1 -- L_72475426/LConn1
  T_72475426_380000_Chiari/RConn2 -- L_72475426/LConn2
  L_72475426/LConn3 -- T_72475426_380000_Chiari/RConn3 -- bus825/LConn1
  T_80399102_380000_Roma_Ovest/RConn1 -- L_80399102/LConn1
  T_80399102_380000_Roma_Ovest/RConn2 -- L_80399102/LConn2
  L_80399102/LConn3 -- T_80399102_380000_Roma_Ovest/RConn3 -- bus826/LConn1
  T_145665799_380000_Brindisi_Nord_380/RConn1 -- L_145665799/LConn1
  T_145665799_380000_Brindisi_Nord_380/RConn2 -- L_145665799/LConn2
  L_145665799/LConn3 -- T_145665799_380000_Brindisi_Nord_380/RConn3 -- bus827/LConn1
  T_132450233_380000_Sparanise/RConn1 -- L_132450233/LConn1
  T_132450233_380000_Sparanise/RConn2 -- L_132450233/LConn2
  L_132450233/LConn3 -- T_132450233_380000_Sparanise/RConn3 -- bus828/LConn1
  T_100407575_380000_Fusina_Termica_sezione_1_400/RConn1 -- L_100407575/LConn1
  T_100407575_380000_Fusina_Termica_sezione_1_400/RConn2 -- L_100407575/LConn2
  L_100407575/LConn3 -- T_100407575_380000_Fusina_Termica_sezione_1_400/RConn3 -- bus829/LConn1
  T_172302572_380000_Aprilia_380/RConn1 -- L_172302572/LConn1
  T_172302572_380000_Aprilia_380/RConn2 -- L_172302572/LConn2
  L_172302572/LConn3 -- T_172302572_380000_Aprilia_380/RConn3 -- bus830/LConn1
  T_42206116_380000_Gorlago/RConn1 -- L_42206116/LConn1
  T_42206116_380000_Gorlago/RConn2 -- L_42206116/LConn2
  L_42206116/LConn3 -- T_42206116_380000_Gorlago/RConn3 -- bus831/LConn1
  T_145665323__/RConn1 -- L_145665323/LConn1
  T_145665323__/RConn2 -- L_145665323/LConn2
  L_145665323/LConn3 -- T_145665323__/RConn3 -- bus832/LConn1
  T_145665862_380000_Enipower_Brindisi_380/RConn1 -- L_145665862/LConn1
  T_145665862_380000_Enipower_Brindisi_380/RConn2 -- L_145665862/LConn2
  L_145665862/LConn3 -- T_145665862_380000_Enipower_Brindisi_380/RConn3 -- bus833/LConn1
  T_414663585_380000_Rosen/RConn1 -- L_414663585/LConn1
  T_414663585_380000_Rosen/RConn2 -- L_414663585/LConn2
  L_414663585/LConn3 -- T_414663585_380000_Rosen/RConn3 -- bus834/LConn1
  T_339104227_380000_Turano_centrale/RConn1 -- L_339104227/LConn1
  T_339104227_380000_Turano_centrale/RConn2 -- L_339104227/LConn2
  L_339104227/LConn3 -- T_339104227_380000_Turano_centrale/RConn3 -- bus835/LConn1
  T_284418385_380000_Stazione_Elettrica_Villafranca_2/RConn1 -- L_284418385/LConn1
  T_284418385_380000_Stazione_Elettrica_Villafranca_2/RConn2 -- L_284418385/LConn2
  L_284418385/LConn3 -- T_284418385_380000_Stazione_Elettrica_Villafranca_2/RConn3 -- bus836/LConn1
  T_110660048__/RConn1 -- L_110660048/LConn1
  T_110660048__/RConn2 -- L_110660048/LConn2
  L_110660048/LConn3 -- T_110660048__/RConn3 -- bus837/LConn1
  T_61157826_380000_Barca___Paternò/RConn1 -- L_61157826/LConn1
  T_61157826_380000_Barca___Paternò/RConn2 -- L_61157826/LConn2
  L_61157826/LConn3 -- T_61157826_380000_Barca___Paternò/RConn3 -- bus838/LConn1
  T_339706878_380000_Ceprano/RConn1 -- L_339706878/LConn1
  T_339706878_380000_Ceprano/RConn2 -- L_339706878/LConn2
  L_339706878/LConn3 -- T_339706878_380000_Ceprano/RConn3 -- bus839/LConn1
  T_155158689_380000_Adria_Sud/RConn1 -- L_155158689/LConn1
  T_155158689_380000_Adria_Sud/RConn2 -- L_155158689/LConn2
  L_155158689/LConn3 -- T_155158689_380000_Adria_Sud/RConn3 -- bus840/LConn1
  T_421827451_380000_La_Casella_centrale/RConn1 -- L_421827451/LConn1
  T_421827451_380000_La_Casella_centrale/RConn2 -- L_421827451/LConn2
  L_421827451/LConn3 -- T_421827451_380000_La_Casella_centrale/RConn3 -- bus841/LConn1
  T_107438024_380000_La_Casella/RConn1 -- L_107438024/LConn1
  T_107438024_380000_La_Casella/RConn2 -- L_107438024/LConn2
  L_107438024/LConn3 -- T_107438024_380000_La_Casella/RConn3 -- bus842/LConn1
  T_421827453_380000_Piacenza/RConn1 -- L_421827453/LConn1
  T_421827453_380000_Piacenza/RConn2 -- L_421827453/LConn2
  L_421827453/LConn3 -- T_421827453_380000_Piacenza/RConn3 -- bus843/LConn1
  T_332123608__/RConn1 -- L_332123608/LConn1
  T_332123608__/RConn2 -- L_332123608/LConn2
  L_332123608/LConn3 -- T_332123608__/RConn3 -- bus844/LConn1
  T_75602396_380000_Pian_Camuno/RConn1 -- L_75602396/LConn1
  T_75602396_380000_Pian_Camuno/RConn2 -- L_75602396/LConn2
  L_75602396/LConn3 -- T_75602396_380000_Pian_Camuno/RConn3 -- bus845/LConn1
  T_116519166_380000_Isp_Cremona/RConn1 -- L_116519166/LConn1
  T_116519166_380000_Isp_Cremona/RConn2 -- L_116519166/LConn2
  L_116519166/LConn3 -- T_116519166_380000_Isp_Cremona/RConn3 -- bus846/LConn1
